simulink model "heart_model"  (R2015a)
settings: Solver=ode3  StartTime=0.0  StopTime=size(sasignal,1)  FixedStep=1  RelTol=1e-6  AbsTol=1e-6
values from neighbouring files (symbols this model uses):
  beta1 = [-1 -0.3 -0.09 -0.3 -0.3 -0.3 -0.3 -0.3 -0.3 -0.3 -0.3 -0.3 ... (33 elements, 1x33)]    [pacemaker_heart_params.mat]
  beta3 = [200 200 200 200 200 200 200 200 200 200 200 200 ... (33 elements, 1x33)]    [pacemaker_heart_params.mat]
  beta4 = [-0.05 -0.05 -0.02 -0.02 -0.02 -0.02 -0.02 -0.02 -0.02 -0.02 -0.02 -0.02 ... (33 elements, 1x33)]    [pacemaker_heart_params.mat]
  delay = [15.5648 23.2106666667 5.18826666667 12.0149333333 12.8341333333 10.9226666667 18.5685333333 9.55733333333 12.8341333333 4.36906666667 5.46133333333 9.8304 ... (34 elements, 1x34)]    [pacemaker_heart_params.mat]
  gain = [0.1 0.1 0.1 0.1 0.07 0.1 0.1 0.1 0.1 0.1 0.1 0.1 ... (33 elements, 1x33)]    [pacemaker_heart_params.mat]
libraries: simulink x40, dspsrcs4 x1
(part 4 of 5)

== system heart_model/Heart Model/VENTRICLE/RVA (15)/Subsystem3/Subsystem ==
  q : Inport
  v : Inport  Port=2
  f(vno) : Inport  Port=3
  vin : Inport  Port=4
  win : Inport  Port=5
  Gain3 : Gain  Gain=-1
  Multiport Switch : MultiPortSwitch  Inputs=4
  Product : Product  RndMeth=Zero
  Product1 : Product  RndMeth=Zero
  Sum : Sum  Inputs=|++
  Sum1 : Sum  Inputs=|++
  beta1 : Gain  Gain=beta1(15)
  beta3 : Gain  Gain=beta3(15)
  beta4 : Gain  Gain=beta4(15)
  vgain : Outport
  wires:
  Gain3/1 -> Product1/2
  Product1/1 -> Multiport Switch/3, Sum1/2
  Sum1/1 -> Multiport Switch/2
  Sum/1 -> Sum1/1
  win/1 -> Gain3/1
  vin/1 -> Sum/1
  beta1/1 -> Sum/2
  f(vno)/1 -> Product/2
  beta4/1 -> Product/1
  Product/1 -> Multiport Switch/5
  v/1 -> Product1/1, beta4/1, beta3/1, beta1/1
  beta3/1 -> Multiport Switch/4
  Multiport Switch/1 -> vgain/1
  q/1 -> Multiport Switch/1

== system heart_model/Heart Model/VENTRICLE/RVA (15)/Subsystem3/Subsystem2 ==
  I_st : Inport
  q : Inport  Port=2
  vgain : Inport  Port=3
  vin : Inport  Port=4
  Compare To Constant : simulink/Logic and Bit Operations/Compare To Constant  relop===  const=2  OutDataTypeStr=uint8
  Sum : Sum  Inputs=|++
  Sum1 : Sum  Inputs=|++
  Switch : Switch  Criteria=u2 ~= 0
  vint : Outport
  wires:
  Sum1/1 -> Switch/1
  Sum/1 -> Sum1/2
  vin/1 -> Sum/2
  I_st/1 -> Sum/1
  vgain/1 -> Sum1/1, Switch/3
  Switch/1 -> vint/1
  q/1 -> Compare To Constant/1
  Compare To Constant/1 -> Switch/2

== system heart_model/Heart Model/VENTRICLE/RV_m (17)/Subsystem3/Subsystem ==
  q : Inport
  v : Inport  Port=2
  f(vno) : Inport  Port=3
  vin : Inport  Port=4
  win : Inport  Port=5
  Gain3 : Gain  Gain=-1
  Multiport Switch : MultiPortSwitch  Inputs=4
  Product : Product  RndMeth=Zero
  Product1 : Product  RndMeth=Zero
  Sum : Sum  Inputs=|++
  Sum1 : Sum  Inputs=|++
  beta1 : Gain  Gain=beta1(17)
  beta3 : Gain  Gain=beta3(17)
  beta4 : Gain  Gain=beta4(17)
  vgain : Outport
  wires:
  Gain3/1 -> Product1/2
  Product1/1 -> Multiport Switch/3, Sum1/2
  Sum1/1 -> Multiport Switch/2
  Sum/1 -> Sum1/1
  win/1 -> Gain3/1
  vin/1 -> Sum/1
  beta1/1 -> Sum/2
  f(vno)/1 -> Product/2
  beta4/1 -> Product/1
  Product/1 -> Multiport Switch/5
  v/1 -> Product1/1, beta4/1, beta3/1, beta1/1
  beta3/1 -> Multiport Switch/4
  Multiport Switch/1 -> vgain/1
  q/1 -> Multiport Switch/1

== system heart_model/Heart Model/VENTRICLE/RV_m (17)/Subsystem3/Subsystem2 ==
  I_st : Inport
  q : Inport  Port=2
  vgain : Inport  Port=3
  vin : Inport  Port=4
  Compare To Constant : simulink/Logic and Bit Operations/Compare To Constant  relop===  const=2  OutDataTypeStr=uint8
  Sum : Sum  Inputs=|++
  Sum1 : Sum  Inputs=|++
  Switch : Switch  Criteria=u2 ~= 0
  vint : Outport
  wires:
  Sum1/1 -> Switch/1
  Sum/1 -> Sum1/2
  vin/1 -> Sum/2
  I_st/1 -> Sum/1
  vgain/1 -> Sum1/1, Switch/3
  Switch/1 -> vint/1
  q/1 -> Compare To Constant/1
  Compare To Constant/1 -> Switch/2

== system heart_model/Heart Model/VENTRICLE/SEP_LV (27)/Subsystem3/Subsystem ==
  q : Inport
  v : Inport  Port=2
  f(vno) : Inport  Port=3
  vin : Inport  Port=4
  win : Inport  Port=5
  Gain3 : Gain  Gain=-1
  Multiport Switch : MultiPortSwitch  Inputs=4
  Product : Product  RndMeth=Zero
  Product1 : Product  RndMeth=Zero
  Sum : Sum  Inputs=|++
  Sum1 : Sum  Inputs=|++
  beta1 : Gain  Gain=beta1(27)
  beta3 : Gain  Gain=beta3(27)
  beta4 : Gain  Gain=beta4(27)
  vgain : Outport
  wires:
  Gain3/1 -> Product1/2
  Product1/1 -> Multiport Switch/3, Sum1/2
  Sum1/1 -> Multiport Switch/2
  Sum/1 -> Sum1/1
  win/1 -> Gain3/1
  vin/1 -> Sum/1
  beta1/1 -> Sum/2
  f(vno)/1 -> Product/2
  beta4/1 -> Product/1
  Product/1 -> Multiport Switch/5
  v/1 -> Product1/1, beta4/1, beta3/1, beta1/1
  beta3/1 -> Multiport Switch/4
  Multiport Switch/1 -> vgain/1
  q/1 -> Multiport Switch/1

== system heart_model/Heart Model/VENTRICLE/SEP_LV (27)/Subsystem3/Subsystem2 ==
  I_st : Inport
  q : Inport  Port=2
  vgain : Inport  Port=3
  vin : Inport  Port=4
  Compare To Constant : simulink/Logic and Bit Operations/Compare To Constant  relop===  const=2  OutDataTypeStr=uint8
  Sum : Sum  Inputs=|++
  Sum1 : Sum  Inputs=|++
  Switch : Switch  Criteria=u2 ~= 0
  vint : Outport
  wires:
  Sum1/1 -> Switch/1
  Sum/1 -> Sum1/2
  vin/1 -> Sum/2
  I_st/1 -> Sum/1
  vgain/1 -> Sum1/1, Switch/3
  Switch/1 -> vint/1
  q/1 -> Compare To Constant/1
  Compare To Constant/1 -> Switch/2

== system heart_model/Heart Model/VENTRICLE/SEP_LV_m (26)/Subsystem3/Subsystem ==
  q : Inport
  v : Inport  Port=2
  f(vno) : Inport  Port=3
  vin : Inport  Port=4
  win : Inport  Port=5
  Gain3 : Gain  Gain=-1
  Multiport Switch : MultiPortSwitch  Inputs=4
  Product : Product  RndMeth=Zero
  Product1 : Product  RndMeth=Zero
  Sum : Sum  Inputs=|++
  Sum1 : Sum  Inputs=|++
  beta1 : Gain  Gain=beta1(26)
  beta3 : Gain  Gain=beta3(26)
  beta4 : Gain  Gain=beta4(26)
  vgain : Outport
  wires:
  Gain3/1 -> Product1/2
  Product1/1 -> Multiport Switch/3, Sum1/2
  Sum1/1 -> Multiport Switch/2
  Sum/1 -> Sum1/1
  win/1 -> Gain3/1
  vin/1 -> Sum/1
  beta1/1 -> Sum/2
  f(vno)/1 -> Product/2
  beta4/1 -> Product/1
  Product/1 -> Multiport Switch/5
  v/1 -> Product1/1, beta4/1, beta3/1, beta1/1
  beta3/1 -> Multiport Switch/4
  Multiport Switch/1 -> vgain/1
  q/1 -> Multiport Switch/1

== system heart_model/Heart Model/VENTRICLE/SEP_LV_m (26)/Subsystem3/Subsystem2 ==
  I_st : Inport
  q : Inport  Port=2
  vgain : Inport  Port=3
  vin : Inport  Port=4
  Compare To Constant : simulink/Logic and Bit Operations/Compare To Constant  relop===  const=2  OutDataTypeStr=uint8
  Sum : Sum  Inputs=|++
  Sum1 : Sum  Inputs=|++
  Switch : Switch  Criteria=u2 ~= 0
  vint : Outport
  wires:
  Sum1/1 -> Switch/1
  Sum/1 -> Sum1/2
  vin/1 -> Sum/2
  I_st/1 -> Sum/1
  vgain/1 -> Sum1/1, Switch/3
  Switch/1 -> vint/1
  q/1 -> Compare To Constant/1
  Compare To Constant/1 -> Switch/2

== system heart_model/Heart Model/VENTRICLE/SEP_RV (25)/Subsystem3/Subsystem ==
  q : Inport
  v : Inport  Port=2
  f(vno) : Inport  Port=3
  vin : Inport  Port=4
  win : Inport  Port=5
  Gain3 : Gain  Gain=-1
  Multiport Switch : MultiPortSwitch  Inputs=4
  Product : Product  RndMeth=Zero
  Product1 : Product  RndMeth=Zero
  Sum : Sum  Inputs=|++
  Sum1 : Sum  Inputs=|++
  beta1 : Gain  Gain=beta1(25)
  beta3 : Gain  Gain=beta3(25)
  beta4 : Gain  Gain=beta4(25)
  vgain : Outport
  wires:
  Gain3/1 -> Product1/2
  Product1/1 -> Multiport Switch/3, Sum1/2
  Sum1/1 -> Multiport Switch/2
  Sum/1 -> Sum1/1
  win/1 -> Gain3/1
  vin/1 -> Sum/1
  beta1/1 -> Sum/2
  f(vno)/1 -> Product/2
  beta4/1 -> Product/1
  Product/1 -> Multiport Switch/5
  v/1 -> Product1/1, beta4/1, beta3/1, beta1/1
  beta3/1 -> Multiport Switch/4
  Multiport Switch/1 -> vgain/1
  q/1 -> Multiport Switch/1

== system heart_model/Heart Model/VENTRICLE/SEP_RV (25)/Subsystem3/Subsystem2 ==
  I_st : Inport
  q : Inport  Port=2
  vgain : Inport  Port=3
  vin : Inport  Port=4
  Compare To Constant : simulink/Logic and Bit Operations/Compare To Constant  relop===  const=2  OutDataTypeStr=uint8
  Sum : Sum  Inputs=|++
  Sum1 : Sum  Inputs=|++
  Switch : Switch  Criteria=u2 ~= 0
  vint : Outport
  wires:
  Sum1/1 -> Switch/1
  Sum/1 -> Sum1/2
  vin/1 -> Sum/2
  I_st/1 -> Sum/1
  vgain/1 -> Sum1/1, Switch/3
  Switch/1 -> vint/1
  q/1 -> Compare To Constant/1
  Compare To Constant/1 -> Switch/2

== system heart_model/Heart Model/VENTRICLE/SEP_RV_m (24)/Subsystem3/Subsystem ==
  q : Inport
  v : Inport  Port=2
  f(vno) : Inport  Port=3
  vin : Inport  Port=4
  win : Inport  Port=5
  Gain3 : Gain  Gain=-1
  Multiport Switch : MultiPortSwitch  Inputs=4
  Product : Product  RndMeth=Zero
  Product1 : Product  RndMeth=Zero
  Sum : Sum  Inputs=|++
  Sum1 : Sum  Inputs=|++
  beta1 : Gain  Gain=beta1(24)
  beta3 : Gain  Gain=beta3(24)
  beta4 : Gain  Gain=beta4(24)
  vgain : Outport
  wires:
  Gain3/1 -> Product1/2
  Product1/1 -> Multiport Switch/3, Sum1/2
  Sum1/1 -> Multiport Switch/2
  Sum/1 -> Sum1/1
  win/1 -> Gain3/1
  vin/1 -> Sum/1
  beta1/1 -> Sum/2
  f(vno)/1 -> Product/2
  beta4/1 -> Product/1
  Product/1 -> Multiport Switch/5
  v/1 -> Product1/1, beta4/1, beta3/1, beta1/1
  beta3/1 -> Multiport Switch/4
  Multiport Switch/1 -> vgain/1
  q/1 -> Multiport Switch/1

== system heart_model/Heart Model/VENTRICLE/SEP_RV_m (24)/Subsystem3/Subsystem2 ==
  I_st : Inport
  q : Inport  Port=2
  vgain : Inport  Port=3
  vin : Inport  Port=4
  Compare To Constant : simulink/Logic and Bit Operations/Compare To Constant  relop===  const=2  OutDataTypeStr=uint8
  Sum : Sum  Inputs=|++
  Sum1 : Sum  Inputs=|++
  Switch : Switch  Criteria=u2 ~= 0
  vint : Outport
  wires:
  Sum1/1 -> Switch/1
  Sum/1 -> Sum1/2
  vin/1 -> Sum/2
  I_st/1 -> Sum/1
  vgain/1 -> Sum1/1, Switch/3
  Switch/1 -> vint/1
  q/1 -> Compare To Constant/1
  Compare To Constant/1 -> Switch/2

== stateflow chart heart_model/Heart Model/ATRIUM/Bach (8)/Event generator ==
  settings: sampleTime=inf
  state state
  (default) -> ? [order 1]
  (default) -> state [order 1]
  state -> state [order 3] : [v>=138]/
      | event3;
  state -> state [order 1] : [v<20]/event1;
  state -> state [order 2] : [v>=20&&v<138]/event2;
  data: v input double =0
  events: event1 output EITHER_EDGE_EVENT; event2 output EITHER_EDGE_EVENT; event3 output EITHER_EDGE_EVENT

== stateflow chart heart_model/Heart Model/ATRIUM/Bach (8)/Hybrid set ==
  settings: sampleTime=inf
  state resting/
    entry:q=1;
  state stimulated/
    entry:q=2;
  state plateau/
    entry:q=4;
    vno=vn;
  state upstroke/
    entry:q=3;
  (default) -> ? [order 1]
  stimulated -> resting [order 2] : endpstim/vreset=v;reset;
  (default) -> resting [order 1]
  resting -> stimulated [order 1] : pstim/vreset=v;
      | vn=v;reset;
  resting -> upstroke [order 2] : event2/
      | vreset=v;reset;
  stimulated -> upstroke [order 1] : event2/
      | vreset=v;reset;
  plateau -> resting : event1/
      | vreset=v;reset;
  upstroke -> plateau : event3/
      | vreset=v;reset;
  data: q output double size=1 [1..4] =1; vreset output double =0; v input double size=1; vn local double =0; vno output double =0
  events: event1 input EITHER_EDGE_EVENT; reset output EITHER_EDGE_EVENT; event2 input EITHER_EDGE_EVENT; event3 input EITHER_EDGE_EVENT; pstim input RISING_EDGE_EVENT; endpstim input FALLING_EDGE_EVENT

== stateflow chart heart_model/Heart Model/ATRIUM/CS_LA (29)/Event generator ==
  settings: sampleTime=inf
  state state
  (default) -> ? [order 1]
  (default) -> state [order 1]
  state -> state [order 3] : [v>=138]/
      | event3;
  state -> state [order 1] : [v<20]/event1;
  state -> state [order 2] : [v>=20&&v<138]/event2;
  data: v input double =0
  events: event1 output EITHER_EDGE_EVENT; event2 output EITHER_EDGE_EVENT; event3 output EITHER_EDGE_EVENT

== stateflow chart heart_model/Heart Model/ATRIUM/CS_LA (29)/Hybrid set ==
  settings: sampleTime=inf
  state resting/
    entry:q=1;
  state stimulated/
    entry:q=2;
  state plateau/
    entry:q=4;
    vno=vn;
  state upstroke/
    entry:q=3;
  (default) -> ? [order 1]
  stimulated -> resting [order 2] : endpstim/vreset=v;reset;
  (default) -> resting [order 1]
  resting -> stimulated [order 1] : pstim/vreset=v;
      | vn=v;reset;
  resting -> upstroke [order 2] : event2/
      | vreset=v;reset;
  stimulated -> upstroke [order 1] : event2/
      | vreset=v;reset;
  plateau -> resting : event1/
      | vreset=v;reset;
  upstroke -> plateau : event3/
      | vreset=v;reset;
  data: q output double size=1 [1..4] =1; vreset output double =0; v input double size=1; vn local double =0; vno output double =0
  events: event1 input EITHER_EDGE_EVENT; reset output EITHER_EDGE_EVENT; event2 input EITHER_EDGE_EVENT; event3 input EITHER_EDGE_EVENT; pstim input RISING_EDGE_EVENT; endpstim input FALLING_EDGE_EVENT

== stateflow chart heart_model/Heart Model/ATRIUM/CT (2)/Event generator ==
  settings: sampleTime=inf
  state state
  (default) -> ? [order 1]
  (default) -> state [order 1]
  state -> state [order 3] : [v>=138]/
      | event3;
  state -> state [order 1] : [v<20]/event1;
  state -> state [order 2] : [v>=20&&v<138]/event2;
  data: v input double =0
  events: event1 output EITHER_EDGE_EVENT; event2 output EITHER_EDGE_EVENT; event3 output EITHER_EDGE_EVENT

== stateflow chart heart_model/Heart Model/ATRIUM/CT (2)/Hybrid set ==
  settings: sampleTime=inf
  state resting/
    entry:q=1;
  state stimulated/
    entry:q=2;
  state plateau/
    entry:q=4;
    vno=vn;
  state upstroke/
    entry:q=3;
  (default) -> ? [order 1]
  stimulated -> resting [order 2] : endpstim/vreset=v;reset;
  (default) -> resting [order 1]
  resting -> stimulated [order 1] : pstim/vreset=v;
      | vn=v;reset;
  resting -> upstroke [order 2] : event2/
      | vreset=v;reset;
  stimulated -> upstroke [order 1] : event2/
      | vreset=v;reset;
  plateau -> resting : event1/
      | vreset=v;reset;
  upstroke -> plateau : event3/
      | vreset=v;reset;
  data: q output double size=1 [1..4] =1; vreset output double =0; v input double size=1; vn local double =0; vno output double =0
  events: event1 input EITHER_EDGE_EVENT; reset output EITHER_EDGE_EVENT; event2 input EITHER_EDGE_EVENT; event3 input EITHER_EDGE_EVENT; pstim input RISING_EDGE_EVENT; endpstim input FALLING_EDGE_EVENT

== stateflow chart heart_model/Heart Model/ATRIUM/CT_a (21)/Event generator ==
  settings: sampleTime=inf
  state state
  (default) -> ? [order 1]
  (default) -> state [order 1]
  state -> state [order 3] : [v>=138]/
      | event3;
  state -> state [order 1] : [v<20]/event1;
  state -> state [order 2] : [v>=20&&v<138]/event2;
  data: v input double =0
  events: event1 output EITHER_EDGE_EVENT; event2 output EITHER_EDGE_EVENT; event3 output EITHER_EDGE_EVENT

== stateflow chart heart_model/Heart Model/ATRIUM/CT_a (21)/Hybrid set ==
  settings: sampleTime=inf
  state stimulated/
    entry:q=2;
  state resting/
    entry:q=1;
  state plateau/
    entry:q=4;
    vno=vn;
  state upstroke/
    entry:q=3;
  stimulated -> resting [order 1] : endpstim/vreset=v;reset;
  (default) -> resting
  resting -> stimulated [order 1] : pstim/vreset=v;
      | vn=v;reset;
  resting -> upstroke [order 2] : event2/
      | vreset=v;reset;
  stimulated -> upstroke [order 2] : event2/
      | vreset=v;reset;
  plateau -> resting : event1/
      | vreset=v;reset;
  upstroke -> plateau : event3/
      | vreset=v;reset;
  data: q output double size=1 [1..4] =1; vreset output double =0; v input double size=1; vn local double =0; vno output double =0
  events: event1 input EITHER_EDGE_EVENT; reset output EITHER_EDGE_EVENT; event2 input EITHER_EDGE_EVENT; event3 input EITHER_EDGE_EVENT; pstim input RISING_EDGE_EVENT; endpstim input FALLING_EDGE_EVENT

== stateflow chart heart_model/Heart Model/ATRIUM/Fast (32)/Event generator ==
  settings: sampleTime=inf
  state state
  (default) -> ? [order 1]
  (default) -> state [order 1]
  state -> state [order 3] : [v>=138]/
      | event3;
  state -> state [order 1] : [v<20]/event1;
  state -> state [order 2] : [v>=20&&v<138]/event2;
  data: v input double =0
  events: event1 output EITHER_EDGE_EVENT; event2 output EITHER_EDGE_EVENT; event3 output EITHER_EDGE_EVENT

== stateflow chart heart_model/Heart Model/ATRIUM/Fast (32)/Hybrid set ==
  settings: sampleTime=inf
  state resting/
    entry:q=1;
  state stimulated/
    entry:q=2;
  state plateau/
    entry:q=4;
    vno=vn;
  state upstroke/
    entry:q=3;
  (default) -> ? [order 1]
  stimulated -> resting [order 2] : endpstim/vreset=v;reset;
  (default) -> resting [order 1]
  resting -> stimulated [order 1] : pstim/vreset=v;
      | vn=v;reset;
  resting -> upstroke [order 2] : event2/
      | vreset=v;reset;
  stimulated -> upstroke [order 1] : event2/
      | vreset=v;reset;
  plateau -> resting : event1/
      | vreset=v;reset;
  upstroke -> plateau : event3/
      | vreset=v;reset;
  data: q output double size=1 [1..4] =1; vreset output double =0; v input double size=1; vn local double =0; vno output double =0
  events: event1 input EITHER_EDGE_EVENT; reset output EITHER_EDGE_EVENT; event2 input EITHER_EDGE_EVENT; event3 input EITHER_EDGE_EVENT; pstim input RISING_EDGE_EVENT; endpstim input FALLING_EDGE_EVENT

== stateflow chart heart_model/Heart Model/ATRIUM/Fast_b (33)/Event generator ==
  settings: sampleTime=inf
  state state
  (default) -> ? [order 1]
  (default) -> state [order 1]
  state -> state [order 3] : [v>=138]/
      | event3;
  state -> state [order 1] : [v<20]/event1;
  state -> state [order 2] : [v>=20&&v<138]/event2;
  data: v input double =0
  events: event1 output EITHER_EDGE_EVENT; event2 output EITHER_EDGE_EVENT; event3 output EITHER_EDGE_EVENT

== stateflow chart heart_model/Heart Model/ATRIUM/Fast_b (33)/Hybrid set ==
  settings: sampleTime=inf
  state resting/
    entry:q=1;
  state stimulated/
    entry:q=2;
  state plateau/
    entry:q=4;
    vno=vn;
  state upstroke/
    entry:q=3;
  (default) -> ? [order 1]
  stimulated -> resting [order 2] : endpstim/vreset=v;reset;
  (default) -> resting [order 1]
  resting -> stimulated [order 1] : pstim/vreset=v;
      | vn=v;reset;
  resting -> upstroke [order 2] : event2/
      | vreset=v;reset;
  stimulated -> upstroke [order 1] : event2/
      | vreset=v;reset;
  plateau -> resting : event1/
      | vreset=v;reset;
  upstroke -> plateau : event3/
      | vreset=v;reset;
  data: q output double size=1 [1..4] =1; vreset output double =0; v input double size=1; vn local double =0; vno output double =0
  events: event1 input EITHER_EDGE_EVENT; reset output EITHER_EDGE_EVENT; event2 input EITHER_EDGE_EVENT; event3 input EITHER_EDGE_EVENT; pstim input RISING_EDGE_EVENT; endpstim input FALLING_EDGE_EVENT

== stateflow chart heart_model/Heart Model/ATRIUM/LA (10)/Event generator ==
  settings: sampleTime=inf
  state state
  (default) -> ? [order 1]
  (default) -> state [order 1]
  state -> state [order 3] : [v>=138]/
      | event3;
  state -> state [order 1] : [v<20]/event1;
  state -> state [order 2] : [v>=20&&v<138]/event2;
  data: v input double =0
  events: event1 output EITHER_EDGE_EVENT; event2 output EITHER_EDGE_EVENT; event3 output EITHER_EDGE_EVENT

== stateflow chart heart_model/Heart Model/ATRIUM/LA (10)/Hybrid set ==
  settings: sampleTime=inf
  state resting/
    entry:q=1;
  state stimulated/
    entry:q=2;
  state plateau/
    entry:q=4;
    vno=vn;
  state upstroke/
    entry:q=3;
  (default) -> ? [order 1]
  stimulated -> resting [order 2] : endpstim/vreset=v;reset;
  (default) -> resting [order 1]
  resting -> stimulated [order 1] : pstim/vreset=v;
      | vn=v;reset;
  resting -> upstroke [order 2] : event2/
      | vreset=v;reset;
  stimulated -> upstroke [order 1] : event2/
      | vreset=v;reset;
  plateau -> resting : event1/
      | vreset=v;reset;
  upstroke -> plateau : event3/
      | vreset=v;reset;
  data: q output double size=1 [1..4] =1; vreset output double =0; v input double size=1; vn local double =0; vno output double =0
  events: event1 input EITHER_EDGE_EVENT; reset output EITHER_EDGE_EVENT; event2 input EITHER_EDGE_EVENT; event3 input EITHER_EDGE_EVENT; pstim input RISING_EDGE_EVENT; endpstim input FALLING_EDGE_EVENT

== stateflow chart heart_model/Heart Model/ATRIUM/LA_a (9)/Event generator ==
  settings: sampleTime=inf
  state state
  (default) -> ? [order 1]
  (default) -> state [order 1]
  state -> state [order 3] : [v>=138]/
      | event3;
  state -> state [order 1] : [v<20]/event1;
  state -> state [order 2] : [v>=20&&v<138]/event2;
  data: v input double =0
  events: event1 output EITHER_EDGE_EVENT; event2 output EITHER_EDGE_EVENT; event3 output EITHER_EDGE_EVENT

== stateflow chart heart_model/Heart Model/ATRIUM/LA_a (9)/Hybrid set ==
  settings: sampleTime=inf
  state resting/
    entry:q=1;
  state stimulated/
    entry:q=2;
  state plateau/
    entry:q=4;
    vno=vn;
  state upstroke/
    entry:q=3;
  (default) -> ? [order 1]
  stimulated -> resting [order 2] : endpstim/vreset=v;reset;
  (default) -> resting [order 1]
  resting -> stimulated [order 1] : pstim/vreset=v;
      | vn=v;reset;
  resting -> upstroke [order 2] : event2/
      | vreset=v;reset;
  stimulated -> upstroke [order 1] : event2/
      | vreset=v;reset;
  plateau -> resting : event1/
      | vreset=v;reset;
  upstroke -> plateau : event3/
      | vreset=v;reset;
  data: q output double size=1 [1..4] =1; vreset output double =0; v input double size=1; vn local double =0; vno output double =0
  events: event1 input EITHER_EDGE_EVENT; reset output EITHER_EDGE_EVENT; event2 input EITHER_EDGE_EVENT; event3 input EITHER_EDGE_EVENT; pstim input RISING_EDGE_EVENT; endpstim input FALLING_EDGE_EVENT

== stateflow chart heart_model/Heart Model/ATRIUM/OS (4)/Event generator ==
  settings: sampleTime=inf
  state state
  (default) -> ? [order 1]
  (default) -> state [order 1]
  state -> state [order 3] : [v>=138]/
      | event3;
  state -> state [order 1] : [v<20]/event1;
  state -> state [order 2] : [v>=20&&v<138]/event2;
  data: v input double =0
  events: event1 output EITHER_EDGE_EVENT; event2 output EITHER_EDGE_EVENT; event3 output EITHER_EDGE_EVENT

== stateflow chart heart_model/Heart Model/ATRIUM/OS (4)/Hybrid set ==
  settings: sampleTime=inf
  state resting/
    entry:q=1;
  state stimulated/
    entry:q=2;
  state plateau/
    entry:q=4;
    vno=vn;
  state upstroke/
    entry:q=3;
  (default) -> ? [order 1]
  stimulated -> resting [order 2] : endpstim/vreset=v;reset;
  (default) -> resting [order 1]
  resting -> stimulated [order 1] : pstim/vreset=v;
      | vn=v;reset;
  resting -> upstroke [order 2] : event2/
      | vreset=v;reset;
  stimulated -> upstroke [order 1] : event2/
      | vreset=v;reset;
  plateau -> resting : event1/
      | vreset=v;reset;
  upstroke -> plateau : event3/
      | vreset=v;reset;
  data: q output double size=1 [1..4] =1; vreset output double =0; v input double size=1; vn local double =0; vno output double =0
  events: event1 input EITHER_EDGE_EVENT; reset output EITHER_EDGE_EVENT; event2 input EITHER_EDGE_EVENT; event3 input EITHER_EDGE_EVENT; pstim input RISING_EDGE_EVENT; endpstim input FALLING_EDGE_EVENT

== stateflow chart heart_model/Heart Model/ATRIUM/RA (23)/Event generator ==
  settings: sampleTime=inf
  state state
  (default) -> ? [order 1]
  (default) -> state [order 1]
  state -> state [order 3] : [v>=138]/
      | event3;
  state -> state [order 1] : [v<20]/event1;
  state -> state [order 2] : [v>=20&&v<138]/event2;
  data: v input double =0
  events: event1 output EITHER_EDGE_EVENT; event2 output EITHER_EDGE_EVENT; event3 output EITHER_EDGE_EVENT

== stateflow chart heart_model/Heart Model/ATRIUM/RA (23)/Hybrid set ==
  settings: sampleTime=inf
  state resting/
    entry:q=1;
  state stimulated/
    entry:q=2;
  state plateau/
    entry:q=4;
    vno=vn;
  state upstroke/
    entry:q=3;
  (default) -> ? [order 1]
  stimulated -> resting [order 2] : endpstim/vreset=v;reset;
  (default) -> resting [order 1]
  resting -> stimulated [order 1] : pstim/vreset=v;
      | vn=v;reset;
  resting -> upstroke [order 2] : event2/
      | vreset=v;reset;
  stimulated -> upstroke [order 1] : event2/
      | vreset=v;reset;
  plateau -> resting : event1/
      | vreset=v;reset;
  upstroke -> plateau : event3/
      | vreset=v;reset;
  data: q output double size=1 [1..4] =1; vreset output double =0; v input double size=1; vn local double =0; vno output double =0
  events: event1 input EITHER_EDGE_EVENT; reset output EITHER_EDGE_EVENT; event2 input EITHER_EDGE_EVENT; event3 input EITHER_EDGE_EVENT; pstim input RISING_EDGE_EVENT; endpstim input FALLING_EDGE_EVENT

== stateflow chart heart_model/Heart Model/ATRIUM/RA_a (22)/Event generator ==
  settings: sampleTime=inf
  state state
  (default) -> ? [order 1]
  (default) -> state [order 1]
  state -> state [order 3] : [v>=138]/
      | event3;
  state -> state [order 1] : [v<20]/event1;
  state -> state [order 2] : [v>=20&&v<138]/event2;
  data: v input double =0
  events: event1 output EITHER_EDGE_EVENT; event2 output EITHER_EDGE_EVENT; event3 output EITHER_EDGE_EVENT

== stateflow chart heart_model/Heart Model/ATRIUM/RA_a (22)/Hybrid set ==
  settings: sampleTime=inf
  state resting/
    entry:q=1;
  state stimulated/
    entry:q=2;
  state plateau/
    entry:q=4;
    vno=vn;
  state upstroke/
    entry:q=3;
  (default) -> ? [order 1]
  stimulated -> resting [order 2] : endpstim/vreset=v;reset;
  (default) -> resting [order 1]
  resting -> stimulated [order 1] : pstim/vreset=v;
      | vn=v;reset;
  resting -> upstroke [order 2] : event2/
      | vreset=v;reset;
  stimulated -> upstroke [order 1] : event2/
      | vreset=v;reset;
  plateau -> resting : event1/
      | vreset=v;reset;
  upstroke -> plateau : event3/
      | vreset=v;reset;
  data: q output double size=1 [1..4] =1; vreset output double =0; v input double size=1; vn local double =0; vno output double =0
  events: event1 input EITHER_EDGE_EVENT; reset output EITHER_EDGE_EVENT; event2 input EITHER_EDGE_EVENT; event3 input EITHER_EDGE_EVENT; pstim input RISING_EDGE_EVENT; endpstim input FALLING_EDGE_EVENT

== stateflow chart heart_model/Heart Model/ATRIUM/Slow_a (31)/Event generator ==
  settings: sampleTime=inf
  state state
  (default) -> ? [order 1]
  (default) -> state [order 1]
  state -> state [order 3] : [v>=138]/
      | event3;
  state -> state [order 1] : [v<20]/event1;
  state -> state [order 2] : [v>=20&&v<138]/event2;
  data: v input double =0
  events: event1 output EITHER_EDGE_EVENT; event2 output EITHER_EDGE_EVENT; event3 output EITHER_EDGE_EVENT

== stateflow chart heart_model/Heart Model/ATRIUM/Slow_a (31)/Hybrid set ==
  settings: sampleTime=inf
  state resting/
    entry:q=1;
  state stimulated/
    entry:q=2;
  state plateau/
    entry:q=4;
    vno=vn;
  state upstroke/
    entry:q=3;
  (default) -> ? [order 1]
  stimulated -> resting [order 2] : endpstim/vreset=v;reset;
  (default) -> resting [order 1]
  resting -> stimulated [order 1] : pstim/vreset=v;
      | vn=v;reset;
  resting -> upstroke [order 2] : event2/
      | vreset=v;reset;
  stimulated -> upstroke [order 1] : event2/
      | vreset=v;reset;
  plateau -> resting : event1/
      | vreset=v;reset;
  upstroke -> plateau : event3/
      | vreset=v;reset;
  data: q output double size=1 [1..4] =1; vreset output double =0; v input double size=1; vn local double =0; vno output double =0
  events: event1 input EITHER_EDGE_EVENT; reset output EITHER_EDGE_EVENT; event2 input EITHER_EDGE_EVENT; event3 input EITHER_EDGE_EVENT; pstim input RISING_EDGE_EVENT; endpstim input FALLING_EDGE_EVENT

== stateflow chart heart_model/Heart Model/ATRIUM/Slow_b (30)/Event generator ==
  settings: sampleTime=inf
  state state
  (default) -> ? [order 1]
  (default) -> state [order 1]
  state -> state [order 3] : [v>=138]/
      | event3;
  state -> state [order 1] : [v<20]/event1;
  state -> state [order 2] : [v>=20&&v<138]/event2;
  data: v input double =0
  events: event1 output EITHER_EDGE_EVENT; event2 output EITHER_EDGE_EVENT; event3 output EITHER_EDGE_EVENT

== stateflow chart heart_model/Heart Model/ATRIUM/Slow_b (30)/Hybrid set ==
  settings: sampleTime=inf
  state resting/
    entry:q=1;
  state stimulated/
    entry:q=2;
  state plateau/
    entry:q=4;
    vno=vn;
  state upstroke/
    entry:q=3;
  (default) -> ? [order 1]
  stimulated -> resting [order 2] : endpstim/vreset=v;reset;
  (default) -> resting [order 1]
  resting -> stimulated [order 1] : pstim/vreset=v;
      | vn=v;reset;
  resting -> upstroke [order 2] : event2/
      | vreset=v;reset;
  stimulated -> upstroke [order 1] : event2/
      | vreset=v;reset;
  plateau -> resting : event1/
      | vreset=v;reset;
  upstroke -> plateau : event3/
      | vreset=v;reset;
  data: q output double size=1 [1..4] =1; vreset output double =0; v input double size=1; vn local double =0; vno output double =0
  events: event1 input EITHER_EDGE_EVENT; reset output EITHER_EDGE_EVENT; event2 input EITHER_EDGE_EVENT; event3 input EITHER_EDGE_EVENT; pstim input RISING_EDGE_EVENT; endpstim input FALLING_EDGE_EVENT

== stateflow chart heart_model/Heart Model/AV (3)/Event generator ==
  settings: sampleTime=inf
  state state
  (default) -> ? [order 1]
  (default) -> state [order 1]
  state -> state [order 3] : [v>=138]/
      | event3;
  state -> state [order 1] : [v<20]/event1;
  state -> state [order 2] : [v>=20&&v<138]/event2;
  data: v input double =0
  events: event1 output EITHER_EDGE_EVENT; event2 output EITHER_EDGE_EVENT; event3 output EITHER_EDGE_EVENT

== stateflow chart heart_model/Heart Model/AV (3)/Hybrid set ==
  settings: sampleTime=inf
  state resting/
    entry:q=1;
  state stimulated/
    entry:q=2;
  state plateau/
    entry:q=4;
    vno=vn;
  state upstroke/
    entry:q=3;
  (default) -> ? [order 1]
  stimulated -> resting [order 2] : endpstim/vreset=v;reset;
  (default) -> resting [order 1]
  resting -> stimulated [order 1] : pstim/vreset=v;
      | vn=v;reset;
  resting -> upstroke [order 2] : event2/
      | vreset=v;reset;
  stimulated -> upstroke [order 1] : event2/
      | vreset=v;reset;
  plateau -> resting : event1/
      | vreset=v;reset;
  upstroke -> plateau : event3/
      | vreset=v;reset;
  data: q output double size=1 [1..4] =1; vreset output double =0; v input double size=1; vn local double =0; vno output double =0
  events: event1 input EITHER_EDGE_EVENT; reset output EITHER_EDGE_EVENT; event2 input EITHER_EDGE_EVENT; event3 input EITHER_EDGE_EVENT; pstim input RISING_EDGE_EVENT; endpstim input FALLING_EDGE_EVENT

== stateflow chart heart_model/Heart Model/SA (1)/Event generator ==
  settings: sampleTime=inf
  state state
  (default) -> ? [order 1]
  (default) -> state [order 1]
  state -> state [order 3] : [v>=138]/
      | event3;
  state -> state [order 1] : [v<20]/event1;
  state -> state [order 2] : [v>=20&&v<138]/event2;
  data: v input double =0
  events: event1 output EITHER_EDGE_EVENT; event2 output EITHER_EDGE_EVENT; event3 output EITHER_EDGE_EVENT

== stateflow chart heart_model/Heart Model/SA (1)/Hybrid set ==
  settings: sampleTime=inf
  state resting/
    entry:q=1;
  state stimulated/
    entry:q=2;
  state plateau/
    entry:q=4;
    vno=vn;
  state upstroke/
    entry:q=3;
  (default) -> ? [order 1]
  stimulated -> resting [order 2] : endstim/vreset=v;reset;
  (default) -> resting [order 1]
  resting -> stimulated : stim/vreset=v;
      | vn=v;reset;
  stimulated -> upstroke [order 1] : event2/
      | vreset=v;reset;
  plateau -> resting : event1/
      | vreset=v;reset;
  upstroke -> plateau : event3/
      | vreset=v;reset;
  data: q output double size=1 [1..4] =1; vreset output double =0; v input double size=1; vn local double =0; vno output double =0
  events: event1 input EITHER_EDGE_EVENT; reset output EITHER_EDGE_EVENT; event2 input EITHER_EDGE_EVENT; event3 input EITHER_EDGE_EVENT; stim input RISING_EDGE_EVENT; endstim input FALLING_EDGE_EVENT

== stateflow chart heart_model/Heart Model/VENTRICLE/CS_LV (28)/Event generator ==
  settings: sampleTime=inf
  state state
  (default) -> ? [order 1]
  (default) -> state [order 1]
  state -> state [order 3] : [v>=138]/
      | event3;
  state -> state [order 1] : [v<20]/event1;
  state -> state [order 2] : [v>=20&&v<138]/event2;
  data: v input double =0
  events: event1 output EITHER_EDGE_EVENT; event2 output EITHER_EDGE_EVENT; event3 output EITHER_EDGE_EVENT

== stateflow chart heart_model/Heart Model/VENTRICLE/CS_LV (28)/Hybrid set ==
  settings: sampleTime=inf
  state resting/
    entry:q=1;
  state stimulated/
    entry:q=2;
  state plateau/
    entry:q=4;
    vno=vn;
  state upstroke/
    entry:q=3;
  (default) -> ? [order 1]
  stimulated -> resting [order 2] : endpstim/vreset=v;reset;
  (default) -> resting [order 1]
  resting -> stimulated [order 1] : pstim/vreset=v;
      | vn=v;reset;
  resting -> upstroke [order 2] : event2/
      | vreset=v;reset;
  stimulated -> upstroke [order 1] : event2/
      | vreset=v;reset;
  plateau -> resting : event1/
      | vreset=v;reset;
  upstroke -> plateau : event3/
      | vreset=v;reset;
  data: q output double size=1 [1..4] =1; vreset output double =0; v input double size=1; vn local double =0; vno output double =0
  events: event1 input EITHER_EDGE_EVENT; reset output EITHER_EDGE_EVENT; event2 input EITHER_EDGE_EVENT; event3 input EITHER_EDGE_EVENT; pstim input RISING_EDGE_EVENT; endpstim input FALLING_EDGE_EVENT

== stateflow chart heart_model/Heart Model/VENTRICLE/His_d (7)/Event generator ==
  settings: sampleTime=inf
  state state
  (default) -> ? [order 1]
  (default) -> state [order 1]
  state -> state [order 3] : [v>=138]/
      | event3;
  state -> state [order 1] : [v<20]/event1;
  state -> state [order 2] : [v>=20&&v<138]/event2;
  data: v input double =0
  events: event1 output EITHER_EDGE_EVENT; event2 output EITHER_EDGE_EVENT; event3 output EITHER_EDGE_EVENT

== stateflow chart heart_model/Heart Model/VENTRICLE/His_d (7)/Hybrid set ==
  settings: sampleTime=inf
  state resting/
    entry:q=1;
  state stimulated/
    entry:q=2;
  state plateau/
    entry:q=4;
    vno=vn;
  state upstroke/
    entry:q=3;
  (default) -> ? [order 1]
  stimulated -> resting [order 2] : endpstim/vreset=v;reset;
  (default) -> resting [order 1]
  resting -> stimulated [order 1] : pstim/vreset=v;
      | vn=v;reset;
  resting -> upstroke [order 2] : event2/
      | vreset=v;reset;
  stimulated -> upstroke [order 1] : event2/
      | vreset=v;reset;
  plateau -> resting : event1/
      | vreset=v;reset;
  upstroke -> plateau : event3/
      | vreset=v;reset;
  data: q output double size=1 [1..4] =1; vreset output double =0; v input double size=1; vn local double =0; vno output double =0
  events: event1 input EITHER_EDGE_EVENT; reset output EITHER_EDGE_EVENT; event2 input EITHER_EDGE_EVENT; event3 input EITHER_EDGE_EVENT; pstim input RISING_EDGE_EVENT; endpstim input FALLING_EDGE_EVENT

== stateflow chart heart_model/Heart Model/VENTRICLE/His_m (6)/Event generator ==
  settings: sampleTime=inf
  state state
  (default) -> ? [order 1]
  (default) -> state [order 1]
  state -> state [order 3] : [v>=138]/
      | event3;
  state -> state [order 1] : [v<20]/event1;
  state -> state [order 2] : [v>=20&&v<138]/event2;
  data: v input double =0
  events: event1 output EITHER_EDGE_EVENT; event2 output EITHER_EDGE_EVENT; event3 output EITHER_EDGE_EVENT

== stateflow chart heart_model/Heart Model/VENTRICLE/His_m (6)/Hybrid set ==
  settings: sampleTime=inf
  state resting/
    entry:q=1;
  state stimulated/
    entry:q=2;
  state plateau/
    entry:q=4;
    vno=vn;
  state upstroke/
    entry:q=3;
  (default) -> ? [order 1]
  stimulated -> resting [order 2] : endpstim/vreset=v;reset;
  (default) -> resting [order 1]
  resting -> stimulated [order 1] : pstim/vreset=v;
      | vn=v;reset;
  resting -> upstroke [order 2] : event2/
      | vreset=v;reset;
  stimulated -> upstroke [order 1] : event2/
      | vreset=v;reset;
  plateau -> resting : event1/
      | vreset=v;reset;
  upstroke -> plateau : event3/
      | vreset=v;reset;
  data: q output double size=1 [1..4] =1; vreset output double =0; v input double size=1; vn local double =0; vno output double =0
  events: event1 input EITHER_EDGE_EVENT; reset output EITHER_EDGE_EVENT; event2 input EITHER_EDGE_EVENT; event3 input EITHER_EDGE_EVENT; pstim input RISING_EDGE_EVENT; endpstim input FALLING_EDGE_EVENT

== stateflow chart heart_model/Heart Model/VENTRICLE/His_p (5)/Event generator ==
  settings: sampleTime=inf
  state state
  (default) -> ? [order 1]
  (default) -> state [order 1]
  state -> state [order 3] : [v>=138]/
      | event3;
  state -> state [order 1] : [v<20]/event1;
  state -> state [order 2] : [v>=20&&v<138]/event2;
  data: v input double =0
  events: event1 output EITHER_EDGE_EVENT; event2 output EITHER_EDGE_EVENT; event3 output EITHER_EDGE_EVENT

== stateflow chart heart_model/Heart Model/VENTRICLE/His_p (5)/Hybrid set ==
  settings: sampleTime=inf
  state resting/
    entry:q=1;
  state stimulated/
    entry:q=2;
  state plateau/
    entry:q=4;
    vno=vn;
  state upstroke/
    entry:q=3;
  (default) -> ? [order 1]
  stimulated -> resting [order 2] : endpstim/vreset=v;reset;
  (default) -> resting [order 1]
  resting -> stimulated [order 1] : pstim/vreset=v;
      | vn=v;reset;
  resting -> upstroke [order 2] : event2/
      | vreset=v;reset;
  stimulated -> upstroke [order 1] : event2/
      | vreset=v;reset;
  plateau -> resting : event1/
      | vreset=v;reset;
  upstroke -> plateau : event3/
      | vreset=v;reset;
  data: q output double size=1 [1..4] =1; vreset output double =0; v input double size=1; vn local double =0; vno output double =0
  events: event1 input EITHER_EDGE_EVENT; reset output EITHER_EDGE_EVENT; event2 input EITHER_EDGE_EVENT; event3 input EITHER_EDGE_EVENT; pstim input RISING_EDGE_EVENT; endpstim input FALLING_EDGE_EVENT

== stateflow chart heart_model/Heart Model/VENTRICLE/LBB (14)/Event generator ==
  settings: sampleTime=inf
  state state
  (default) -> ? [order 1]
  (default) -> state [order 1]
  state -> state [order 3] : [v>=138]/
      | event3;
  state -> state [order 1] : [v<20]/event1;
  state -> state [order 2] : [v>=20&&v<138]/event2;
  data: v input double =0
  events: event1 output EITHER_EDGE_EVENT; event2 output EITHER_EDGE_EVENT; event3 output EITHER_EDGE_EVENT

== stateflow chart heart_model/Heart Model/VENTRICLE/LBB (14)/Hybrid set ==
  settings: sampleTime=inf
  state resting/
    entry:q=1;
  state stimulated/
    entry:q=2;
  state plateau/
    entry:q=4;
    vno=vn;
  state upstroke/
    entry:q=3;
  (default) -> ? [order 1]
  stimulated -> resting [order 2] : endpstim/vreset=v;reset;
  (default) -> resting [order 1]
  resting -> stimulated [order 1] : pstim/vreset=v;
      | vn=v;reset;
  resting -> upstroke [order 2] : event2/
      | vreset=v;reset;
  stimulated -> upstroke [order 1] : event2/
      | vreset=v;reset;
  plateau -> resting : event1/
      | vreset=v;reset;
  upstroke -> plateau : event3/
      | vreset=v;reset;
  data: q output double size=1 [1..4] =1; vreset output double =0; v input double size=1; vn local double =0; vno output double =0
  events: event1 input EITHER_EDGE_EVENT; reset output EITHER_EDGE_EVENT; event2 input EITHER_EDGE_EVENT; event3 input EITHER_EDGE_EVENT; pstim input RISING_EDGE_EVENT; endpstim input FALLING_EDGE_EVENT

== stateflow chart heart_model/Heart Model/VENTRICLE/LBB_m (13)/Event generator ==
  settings: sampleTime=inf
  state state
  (default) -> ? [order 1]
  (default) -> state [order 1]
  state -> state [order 3] : [v>=138]/
      | event3;
  state -> state [order 1] : [v<20]/event1;
  state -> state [order 2] : [v>=20&&v<138]/event2;
  data: v input double =0
  events: event1 output EITHER_EDGE_EVENT; event2 output EITHER_EDGE_EVENT; event3 output EITHER_EDGE_EVENT

== stateflow chart heart_model/Heart Model/VENTRICLE/LBB_m (13)/Hybrid set ==
  settings: sampleTime=inf
  state resting/
    entry:q=1;
  state stimulated/
    entry:q=2;
  state plateau/
    entry:q=4;
    vno=vn;
  state upstroke/
    entry:q=3;
  (default) -> ? [order 1]
  stimulated -> resting [order 2] : endpstim/vreset=v;reset;
  (default) -> resting [order 1]
  resting -> stimulated [order 1] : pstim/vreset=v;
      | vn=v;reset;
  resting -> upstroke [order 2] : event2/
      | vreset=v;reset;
  stimulated -> upstroke [order 1] : event2/
      | vreset=v;reset;
  plateau -> resting : event1/
      | vreset=v;reset;
  upstroke -> plateau : event3/
      | vreset=v;reset;
  data: q output double size=1 [1..4] =1; vreset output double =0; v input double size=1; vn local double =0; vno output double =0
  events: event1 input EITHER_EDGE_EVENT; reset output EITHER_EDGE_EVENT; event2 input EITHER_EDGE_EVENT; event3 input EITHER_EDGE_EVENT; pstim input RISING_EDGE_EVENT; endpstim input FALLING_EDGE_EVENT

== stateflow chart heart_model/Heart Model/VENTRICLE/LV (20)/Event generator ==
  settings: sampleTime=inf
  state state
  (default) -> ? [order 1]
  (default) -> state [order 1]
  state -> state [order 3] : [v>=138]/
      | event3;
  state -> state [order 1] : [v<20]/event1;
  state -> state [order 2] : [v>=20&&v<138]/event2;
  data: v input double =0
  events: event1 output EITHER_EDGE_EVENT; event2 output EITHER_EDGE_EVENT; event3 output EITHER_EDGE_EVENT

== stateflow chart heart_model/Heart Model/VENTRICLE/LV (20)/Hybrid set ==
  settings: sampleTime=inf
  state resting/
    entry:q=1;
  state stimulated/
    entry:q=2;
  state plateau/
    entry:q=4;
    vno=vn;
  state upstroke/
    entry:q=3;
  (default) -> ? [order 1]
  stimulated -> resting [order 2] : endpstim/vreset=v;reset;
  (default) -> resting [order 1]
  resting -> stimulated [order 1] : pstim/vreset=v;
      | vn=v;reset;
  resting -> upstroke [order 2] : event2/
      | vreset=v;reset;
  stimulated -> upstroke [order 1] : event2/
      | vreset=v;reset;
  plateau -> resting : event1/
      | vreset=v;reset;
  upstroke -> plateau : event3/
      | vreset=v;reset;
  data: q output double size=1 [1..4] =1; vreset output double =0; v input double size=1; vn local double =0; vno output double =0
  events: event1 input EITHER_EDGE_EVENT; reset output EITHER_EDGE_EVENT; event2 input EITHER_EDGE_EVENT; event3 input EITHER_EDGE_EVENT; pstim input RISING_EDGE_EVENT; endpstim input FALLING_EDGE_EVENT

== stateflow chart heart_model/Heart Model/VENTRICLE/LVA (16)/Event generator ==
  settings: sampleTime=inf
  state state
  (default) -> ? [order 1]
  (default) -> state [order 1]
  state -> state [order 3] : [v>=138]/
      | event3;
  state -> state [order 1] : [v<20]/event1;
  state -> state [order 2] : [v>=20&&v<138]/event2;
  data: v input double =0
  events: event1 output EITHER_EDGE_EVENT; event2 output EITHER_EDGE_EVENT; event3 output EITHER_EDGE_EVENT

== stateflow chart heart_model/Heart Model/VENTRICLE/LVA (16)/Hybrid set ==
  settings: sampleTime=inf
  state resting/
    entry:q=1;
  state stimulated/
    entry:q=2;
  state plateau/
    entry:q=4;
    vno=vn;
  state upstroke/
    entry:q=3;
  (default) -> ? [order 1]
  stimulated -> resting [order 2] : endpstim/vreset=v;reset;
  (default) -> resting [order 1]
  resting -> stimulated [order 1] : pstim/vreset=v;
      | vn=v;reset;
  resting -> upstroke [order 2] : event2/
      | vreset=v;reset;
  stimulated -> upstroke [order 1] : event2/
      | vreset=v;reset;
  plateau -> resting : event1/
      | vreset=v;reset;
  upstroke -> plateau : event3/
      | vreset=v;reset;
  data: q output double size=1 [1..4] =1; vreset output double =0; v input double size=1; vn local double =0; vno output double =0
  events: event1 input EITHER_EDGE_EVENT; reset output EITHER_EDGE_EVENT; event2 input EITHER_EDGE_EVENT; event3 input EITHER_EDGE_EVENT; pstim input RISING_EDGE_EVENT; endpstim input FALLING_EDGE_EVENT

== stateflow chart heart_model/Heart Model/VENTRICLE/LV_m (19)/Event generator ==
  settings: sampleTime=inf
  state state
  (default) -> ? [order 1]
  (default) -> state [order 1]
  state -> state [order 3] : [v>=138]/
      | event3;
  state -> state [order 1] : [v<20]/event1;
  state -> state [order 2] : [v>=20&&v<138]/event2;
  data: v input double =0
  events: event1 output EITHER_EDGE_EVENT; event2 output EITHER_EDGE_EVENT; event3 output EITHER_EDGE_EVENT

== stateflow chart heart_model/Heart Model/VENTRICLE/LV_m (19)/Hybrid set ==
  settings: sampleTime=inf
  state resting/
    entry:q=1;
  state stimulated/
    entry:q=2;
  state plateau/
    entry:q=4;
    vno=vn;
  state upstroke/
    entry:q=3;
  (default) -> ? [order 1]
  stimulated -> resting [order 2] : endpstim/vreset=v;reset;
  (default) -> resting [order 1]
  resting -> stimulated [order 1] : pstim/vreset=v;
      | vn=v;reset;
  resting -> upstroke [order 2] : event2/
      | vreset=v;reset;
  stimulated -> upstroke [order 1] : event2/
      | vreset=v;reset;
  plateau -> resting : event1/
      | vreset=v;reset;
  upstroke -> plateau : event3/
      | vreset=v;reset;
  data: q output double size=1 [1..4] =1; vreset output double =0; v input double size=1; vn local double =0; vno output double =0
  events: event1 input EITHER_EDGE_EVENT; reset output EITHER_EDGE_EVENT; event2 input EITHER_EDGE_EVENT; event3 input EITHER_EDGE_EVENT; pstim input RISING_EDGE_EVENT; endpstim input FALLING_EDGE_EVENT

== stateflow chart heart_model/Heart Model/VENTRICLE/RBB (12)/Event generator ==
  settings: sampleTime=inf
  state state
  (default) -> ? [order 1]
  (default) -> state [order 1]
  state -> state [order 3] : [v>=138]/
      | event3;
  state -> state [order 1] : [v<20]/event1;
  state -> state [order 2] : [v>=20&&v<138]/event2;
  data: v input double =0
  events: event1 output EITHER_EDGE_EVENT; event2 output EITHER_EDGE_EVENT; event3 output EITHER_EDGE_EVENT

== stateflow chart heart_model/Heart Model/VENTRICLE/RBB (12)/Hybrid set ==
  settings: sampleTime=inf
  state resting/
    entry:q=1;
  state stimulated/
    entry:q=2;
  state plateau/
    entry:q=4;
    vno=vn;
  state upstroke/
    entry:q=3;
  (default) -> ? [order 1]
  stimulated -> resting [order 2] : endpstim/vreset=v;reset;
  (default) -> resting [order 1]
  resting -> stimulated [order 1] : pstim/vreset=v;
      | vn=v;reset;
  resting -> upstroke [order 2] : event2/
      | vreset=v;reset;
  stimulated -> upstroke [order 1] : event2/
      | vreset=v;reset;
  plateau -> resting : event1/
      | vreset=v;reset;
  upstroke -> plateau : event3/
      | vreset=v;reset;
  data: q output double size=1 [1..4] =1; vreset output double =0; v input double size=1; vn local double =0; vno output double =0
  events: event1 input EITHER_EDGE_EVENT; reset output EITHER_EDGE_EVENT; event2 input EITHER_EDGE_EVENT; event3 input EITHER_EDGE_EVENT; pstim input RISING_EDGE_EVENT; endpstim input FALLING_EDGE_EVENT

== stateflow chart heart_model/Heart Model/VENTRICLE/RBB_m (11)/Event generator ==
  settings: sampleTime=inf
  state state
  (default) -> ? [order 1]
  (default) -> state [order 1]
  state -> state [order 3] : [v>=138]/
      | event3;
  state -> state [order 1] : [v<20]/event1;
  state -> state [order 2] : [v>=20&&v<138]/event2;
  data: v input double =0
  events: event1 output EITHER_EDGE_EVENT; event2 output EITHER_EDGE_EVENT; event3 output EITHER_EDGE_EVENT

== stateflow chart heart_model/Heart Model/VENTRICLE/RBB_m (11)/Hybrid set ==
  settings: sampleTime=inf
  state resting/
    entry:q=1;
  state stimulated/
    entry:q=2;
  state plateau/
    entry:q=4;
    vno=vn;
  state upstroke/
    entry:q=3;
  (default) -> ? [order 1]
  stimulated -> resting [order 2] : endpstim/vreset=v;reset;
  (default) -> resting [order 1]
  resting -> stimulated [order 1] : pstim/vreset=v;
      | vn=v;reset;
  resting -> upstroke [order 2] : event2/
      | vreset=v;reset;
  stimulated -> upstroke [order 1] : event2/
      | vreset=v;reset;
  plateau -> resting : event1/
      | vreset=v;reset;
  upstroke -> plateau : event3/
      | vreset=v;reset;
  data: q output double size=1 [1..4] =1; vreset output double =0; v input double size=1; vn local double =0; vno output double =0
  events: event1 input EITHER_EDGE_EVENT; reset output EITHER_EDGE_EVENT; event2 input EITHER_EDGE_EVENT; event3 input EITHER_EDGE_EVENT; pstim input RISING_EDGE_EVENT; endpstim input FALLING_EDGE_EVENT

== stateflow chart heart_model/Heart Model/VENTRICLE/RV (18)/Event generator ==
  settings: sampleTime=inf
  state state
  (default) -> ? [order 1]
  (default) -> state [order 1]
  state -> state [order 3] : [v>=138]/
      | event3;
  state -> state [order 1] : [v<20]/event1;
  state -> state [order 2] : [v>=20&&v<138]/event2;
  data: v input double =0
  events: event1 output EITHER_EDGE_EVENT; event2 output EITHER_EDGE_EVENT; event3 output EITHER_EDGE_EVENT

== stateflow chart heart_model/Heart Model/VENTRICLE/RV (18)/Hybrid set ==
  settings: sampleTime=inf
  state resting/
    entry:q=1;
  state stimulated/
    entry:q=2;
  state plateau/
    entry:q=4;
    vno=vn;
  state upstroke/
    entry:q=3;
  (default) -> ? [order 1]
  stimulated -> resting [order 2] : endpstim/vreset=v;reset;
  (default) -> resting [order 1]
  resting -> stimulated [order 1] : pstim/vreset=v;
      | vn=v;reset;
  resting -> upstroke [order 2] : event2/
      | vreset=v;reset;
  stimulated -> upstroke [order 1] : event2/
      | vreset=v;reset;
  plateau -> resting : event1/
      | vreset=v;reset;
  upstroke -> plateau : event3/
      | vreset=v;reset;
  data: q output double size=1 [1..4] =1; vreset output double =0; v input double size=1; vn local double =0; vno output double =0
  events: event1 input EITHER_EDGE_EVENT; reset output EITHER_EDGE_EVENT; event2 input EITHER_EDGE_EVENT; event3 input EITHER_EDGE_EVENT; pstim input RISING_EDGE_EVENT; endpstim input FALLING_EDGE_EVENT

== stateflow chart heart_model/Heart Model/VENTRICLE/RVA (15)/Event generator ==
  settings: sampleTime=inf
  state state
  (default) -> ? [order 1]
  (default) -> state [order 1]
  state -> state [order 3] : [v>=138]/
      | event3;
  state -> state [order 1] : [v<20]/event1;
  state -> state [order 2] : [v>=20&&v<138]/event2;
  data: v input double =0
  events: event1 output EITHER_EDGE_EVENT; event2 output EITHER_EDGE_EVENT; event3 output EITHER_EDGE_EVENT

== stateflow chart heart_model/Heart Model/VENTRICLE/RVA (15)/Hybrid set ==
  settings: sampleTime=inf
  state resting/
    entry:q=1;
  state stimulated/
    entry:q=2;
  state plateau/
    entry:q=4;
    vno=vn;
  state upstroke/
    entry:q=3;
  (default) -> ? [order 1]
  stimulated -> resting [order 2] : endpstim/vreset=v;reset;
  (default) -> resting [order 1]
  resting -> stimulated [order 1] : pstim/vreset=v;
      | vn=v;reset;
  resting -> upstroke [order 2] : event2/
      | vreset=v;reset;
  stimulated -> upstroke [order 1] : event2/
      | vreset=v;reset;
  plateau -> resting : event1/
      | vreset=v;reset;
  upstroke -> plateau : event3/
      | vreset=v;reset;
  data: q output double size=1 [1..4] =1; vreset output double =0; v input double size=1; vn local double =0; vno output double =0
  events: event1 input EITHER_EDGE_EVENT; reset output EITHER_EDGE_EVENT; event2 input EITHER_EDGE_EVENT; event3 input EITHER_EDGE_EVENT; pstim input RISING_EDGE_EVENT; endpstim input FALLING_EDGE_EVENT

== stateflow chart heart_model/Heart Model/VENTRICLE/RV_m (17)/Event generator ==
  settings: sampleTime=inf
  state state
  (default) -> ? [order 1]
  (default) -> state [order 1]
  state -> state [order 3] : [v>=138]/
      | event3;
  state -> state [order 1] : [v<20]/event1;
  state -> state [order 2] : [v>=20&&v<138]/event2;
  data: v input double =0
  events: event1 output EITHER_EDGE_EVENT; event2 output EITHER_EDGE_EVENT; event3 output EITHER_EDGE_EVENT

== stateflow chart heart_model/Heart Model/VENTRICLE/RV_m (17)/Hybrid set ==
  settings: sampleTime=inf
  state resting/
    entry:q=1;
  state stimulated/
    entry:q=2;
  state plateau/
    entry:q=4;
    vno=vn;
  state upstroke/
    entry:q=3;
  (default) -> ? [order 1]
  stimulated -> resting [order 2] : endpstim/vreset=v;reset;
  (default) -> resting [order 1]
  resting -> stimulated [order 1] : pstim/vreset=v;
      | vn=v;reset;
  resting -> upstroke [order 2] : event2/
      | vreset=v;reset;
  stimulated -> upstroke [order 1] : event2/
      | vreset=v;reset;
  plateau -> resting : event1/
      | vreset=v;reset;
  upstroke -> plateau : event3/
      | vreset=v;reset;
  data: q output double size=1 [1..4] =1; vreset output double =0; v input double size=1; vn local double =0; vno output double =0
  events: event1 input EITHER_EDGE_EVENT; reset output EITHER_EDGE_EVENT; event2 input EITHER_EDGE_EVENT; event3 input EITHER_EDGE_EVENT; pstim input RISING_EDGE_EVENT; endpstim input FALLING_EDGE_EVENT

== stateflow chart heart_model/Heart Model/VENTRICLE/SEP_LV (27)/Event generator ==
  settings: sampleTime=inf
  state state
  (default) -> ? [order 1]
  (default) -> state [order 1]
  state -> state [order 3] : [v>=138]/
      | event3;
  state -> state [order 1] : [v<20]/event1;
  state -> state [order 2] : [v>=20&&v<138]/event2;
  data: v input double =0
  events: event1 output EITHER_EDGE_EVENT; event2 output EITHER_EDGE_EVENT; event3 output EITHER_EDGE_EVENT
